simulink model "Quadrotor_Model2D_2018a"  (R2018a)
settings: Solver=VariableStepAuto  StartTime=0.0  StopTime=300  RelTol=1e-3
settings Model: Creator=Slu03  LastModifiedBy=Charles
settings DebuggingCC: LibraryContextMissingDiagnostic=warning
settings SFSimCC: SimUseLocalCustomCode=on
settings RTWCC: RTWUseLocalCustomCode=on

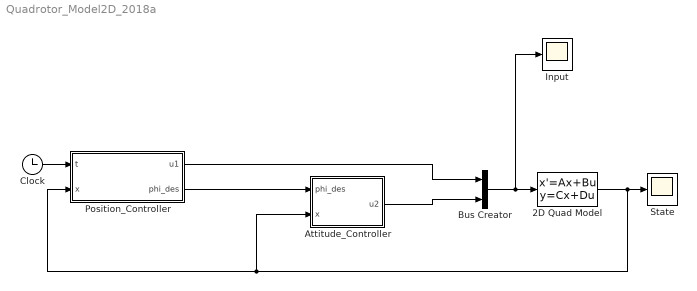
== system Quadrotor_Model2D_2018a ==
  2D Quad Model : StateSpace  A="[zeros(3),eye(3);0 0 -9.8  0 0 0 ;0 0 0 0 0 0;0 0 0 0 0 0]"  B=[zeros(2);zeros(2);33.4 0; 0 10^5/1.43]  C=eye(6)  D=zeros(6,2)  InitialCondition=[2 0 0 0 0 0]
  Attitude_Controller : MATLAB Function  TreatAsAtomicUnit=on
  Bus Creator : BusCreator  Inputs=2
  Clock : Clock
  Input : Scope
  Position_Controller : MATLAB Function  TreatAsAtomicUnit=on
  State : Scope
  wires:
  2D Quad Model/1 -> Position_Controller/2(x), Attitude_Controller/2(x), State/1
  Clock/1 -> Position_Controller/1(t)
  Position_Controller/2(phi_des) -> Attitude_Controller/1(phi_des)
  Bus Creator/1 -> 2D Quad Model/1, Input/1
  Attitude_Controller/1(u2) -> Bus Creator/2
  Position_Controller/1(u1) -> Bus Creator/1

== matlab function Quadrotor_Model2D_2018a/Attitude_Controller ==
  data: phi_des input; u2 output; x input
function u2 = fcn(phi_des,x)

Ixx = 1.43*10^(-5);
kdphi = 4;
kpphi = 4;

phi_ddot = phi_des(3);
phi_dot = phi_des(2);
phi = phi_des(1);

u2 = Ixx*(phi_ddot+kdphi*(phi_dot-x(6))+kpphi*(phi-x(3)));

== matlab function Quadrotor_Model2D_2018a/Position_Controller ==
  data: t input; x input; u1 output; phi_des output
function [u1,phi_des] = fcn(t,x)

% x = [y; z; phi; y_dot; z_dot; phi_dot];
% Here we assume z0 = 0;

y0 = 2;
yh = 5;
zh = 10;
zt = 8;

m = 0.03;
g = 9.8;
kdz = 11;
kpz = 30;
kdy = 4;
kpy = 4;

t1 = 50;
t2 = 100;
T = 100;
t3 = 300;

% Generate the reference
if t<t1
    y = y0;
    y_dot = 0;
    z = zt/t1*t;
    z_dot = zt/t1;
elseif t<t2
    y = y0+(yh-y0)/(t2-t1)*(t-t1);
    y_dot = (yh-y0)/(t2-t1);
    z = zt+(zh-zt)/(t2-t1)*(t-t1);
    z_dot = (zh-zt)/(t2-t1);
elseif t<(t2+T)
    y = yh;
    y_dot = 0;
    z = zh; 
    z_dot = 0;
elseif t<t3
    y = yh;
    y_dot = 0;
    z = zh/(t3-t2-T)*(t3-t);
    z_dot = -zh/(t3-t2-T);
else
    y = yh;
    y_dot = 0;
    z = 0;
    z_dot = 0;
end

phi = -1/g*(kdy*(y_dot-x(4))+kpy*(y-x(1)));
phi_dot = -kdy*x(3)-1/g*kpy*(y_dot-x(4));
u1 = m*(g+kdz*(z_dot-x(5))+kpz*(z-x(2)));
phi_ddot = -kdy*x(6)+kpy*x(3);
phi_des = [phi,phi_dot,phi_ddot];
